simulink library "lib_datainspector_2020a"  (R2020a)
settings: Solver=VariableStepAuto  StartTime=0.0  StopTime=10.0  RelTol=1e-3
libraries: hdlsllib x1
settings Model: Creator=LDM  LastModifiedBy=bin

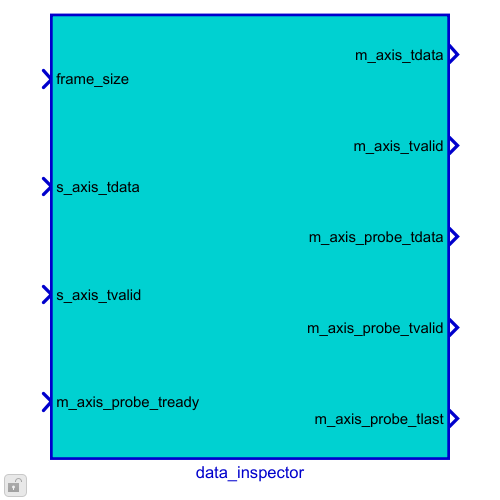
[thumbnail: Simulink's stored preview of the top-level diagram]
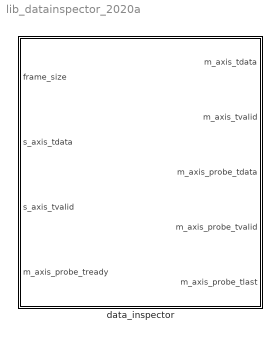
== system lib_datainspector_2020a ==
  data_inspector : Subsystem  TreatAsAtomicUnit=on

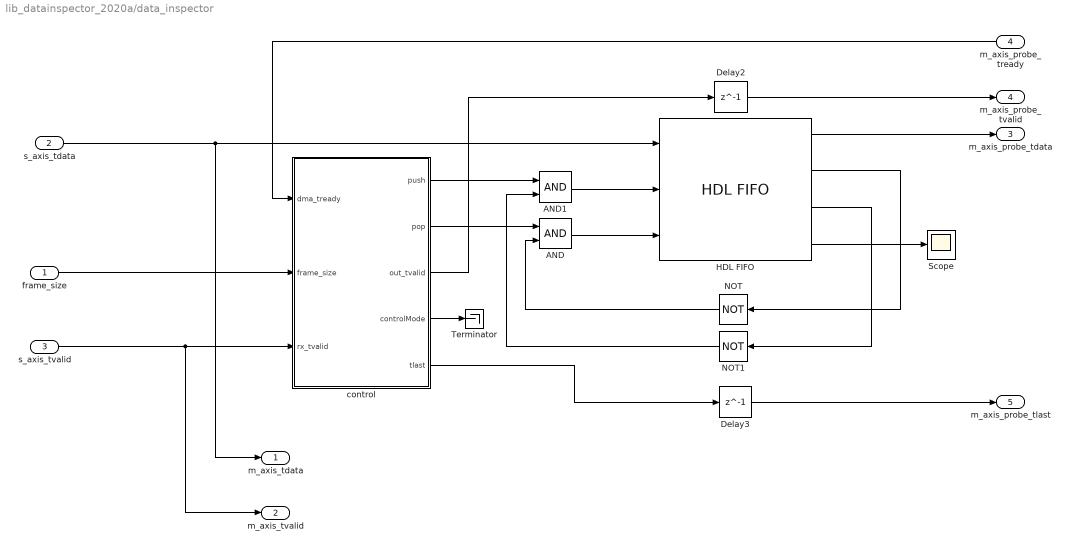
== system lib_datainspector_2020a/data_inspector ==
  frame_size : Inport
  s_axis_tdata : Inport  Port=2
  s_axis_tvalid : Inport  Port=3
  m_axis_probe_tready : Inport  Port=4
  AND : Logic  AllPortsSameDT=off  OutDataTypeStr=boolean
  AND1 : Logic  AllPortsSameDT=off  OutDataTypeStr=boolean
  Delay2 : Delay  DelayLength=1
  Delay3 : Delay  DelayLength=1
  HDL FIFO : hdlsllib/HDL RAMs/HDL FIFO  fifo_size=8192  mode=Classic  ratio=1  push_msg=Warning  pop_msg=Warning  show_empty=on  show_full=on  show_num=on  LabelModeActiveChoice_Mode=Classic  rst_port=off
      settings: SourceProductBaseCode=SL
  NOT : Logic  Operator=NOT  IconShape=distinctive  AllPortsSameDT=off  OutDataTypeStr=boolean
  NOT1 : Logic  Operator=NOT  IconShape=distinctive  AllPortsSameDT=off  OutDataTypeStr=boolean
  Scope : Scope
  Terminator : Terminator
  control : Stateflow chart  TreatAsAtomicUnit=on
  m_axis_tdata : Outport
  m_axis_tvalid : Outport  Port=2
  m_axis_probe_tdata : Outport  Port=3
  m_axis_probe_tvalid : Outport  Port=4
  m_axis_probe_tlast : Outport  Port=5
  wires:
  frame_size/1 -> control/2(frame_size)
  m_axis_probe_tready/1 -> control/1(dma_tready)
  control/2(pop) -> AND/1
  NOT1/1 -> AND1/2
  Delay2/1 -> m_axis_probe_tvalid/1
  control/1(push) -> AND1/1
  HDL FIFO/3 -> NOT1/1
  control/4(controlMode) -> Terminator/1
  AND1/1 -> HDL FIFO/2
  NOT/1 -> AND/2
  s_axis_tdata/1 -> HDL FIFO/1, m_axis_tdata/1
  HDL FIFO/4 -> Scope/1
  AND/1 -> HDL FIFO/3
  control/3(out_tvalid) -> Delay2/1
  HDL FIFO/2 -> NOT/1
  s_axis_tvalid/1 -> m_axis_tvalid/1, control/3(rx_tvalid)
  control/5(tlast) -> Delay3/1
  HDL FIFO/1 -> m_axis_probe_tdata/1
  Delay3/1 -> m_axis_probe_tlast/1

== stateflow chart lib_datainspector_2020a/data_inspector/control ==
  settings: executeAtInitialization=1
  state init
    % variables
    data_count=0;
    % outputs
    push = false
    pop = false
    out_tvalid = false
    tlast = false
  state fill_frame
    % variables
    data_count = data_count + 1
    % outputs
    push = true
    pop = false
    out_tvalid = false
    tlast = false
  state idle1
    % outputs
    push = false
    pop = false
    out_tvalid = false
    tlast = false
  state update
    % outputs
    push = true
    pop = true
    out_tvalid = false
    tlast = false
  state dma_read
    % variables
    data_count = data_count - 1
    % outputs
    push = false
    pop = true
    out_tvalid = true
    tlast = false
  state idle
    % outputs
    push = false
    pop = false
    out_tvalid = false
    tlast = false
  state dma_tlast
    % variables
    data_count = data_count - 1
    % outputs
    push = false
    pop = true
    out_tvalid = true
    tlast = true
  state idle2
    % outputs
    push = false
    pop = false
    out_tvalid = false
    tlast = false
  (default) -> init
  idle1 -> fill_frame [order 1] : [rx_tvalid == true && data_count < frame_size]
  init -> fill_frame : [rx_tvalid == true]
  dma_tlast -> fill_frame [order 2] : [rx_tvalid ==true]
  fill_frame -> dma_read [order 3] : [data_count == frame_size && dma_tready == true]
  fill_frame -> idle1 [order 1] : [rx_tvalid == false]
  fill_frame -> update [order 2] : [data_count == frame_size && dma_tready == false]
  dma_tlast -> idle1 [order 1] : [rx_tvalid == false]
  update -> idle1 [order 2] : [rx_tvalid == false]
  idle1 -> update [order 2] : [rx_tvalid == true && data_count == frame_size]
  update -> dma_read [order 1] : [dma_tready == true]
  dma_read -> idle [order 3] : [dma_tready == false && data_count > 0]
  dma_read -> dma_tlast [order 1] : [data_count == 1 && rx_tvalid ==true]
  idle -> dma_tlast [order 2] : [dma_tready == true && data_count == 1]
  idle -> dma_read [order 1] : [dma_tready == true && data_count > 1]
  dma_read -> idle2 [order 2] : [data_count == 1 && rx_tvalid == false]
  idle2 -> dma_tlast : [dma_tready == true]
  data: dma_tready input boolean; frame_size input; push output boolean; pop output boolean; data_count local uint16; rx_tvalid input; out_tvalid output; controlMode output Enum: controlModeType; tlast output
